simulink model "AOCS_FDIR"  (R2020b)
settings: Solver=ode45  StartTime=0.0  StopTime=200  FixedStep=1e-4  MaxStep=0.25  RelTol=1e-8  AbsTol=1e-8
values from neighbouring files (symbols this model uses):
  Gyros = zeros(3,6)    [Generate_Data.m]
  ReWhe = zeros(3,4)    [Generate_Data.m]
  Thrus = ones(1,8)    [Generate_Data.m]
undefined symbols (not defined in the file or in its folder): A, A_FEEP, A_FEEP_real, A_mag, CG_real, d_face, Dipole_SC, e0_0, e1_0, e2_0, e3_0, e_max_att, e_max_orb, Env_Drag, Env_J2, Env_Moon, Env_Sun, Env_TGG, Env_TMag, FEEP, g, GNSS, gyr, h_ref, h_RW, h_rw_0, I, I_real, IAU, initial_date_JD, J2, K_det, k_quat, km, m, mag, mu, mu_Moon, mu_Sun, n, n_orbits, q_0, Re, RW1, RW2, RW3, RW4, rx0, ry0, rz0, s, sigma1, sigma2, star, T_friction, th_2_gyr, th_FR_gyr, th_RW, th_SD_gyr_null, th_thruster ... (+10)
libraries: dspstat3 x16, aerolibutil x8, sharedutil x6, sharedtransform x5, vrlib x3, aerolibtransform2 x3, aerolibcelestial x2, aerolibobsolete x1, dspinverses x1
(part 1 of 4)
settings Model: PacingRate=1000  Creator=JavierSanzLobo  LastModifiedBy=Pepe
settings SolverCC: AutoScaleAbsTol=off  ShapePreserveControl=EnableAll  ZeroCrossControl=DisableAll  ZeroCrossAlgorithm=Adaptive  AutoInsertRateTranBlk=on  DecoupledContinuousIntegration=on  MinimalZcImpactIntegration=on
settings DataIOCC: ReturnWorkspaceOutputs=off
settings DebuggingCC: ArithmeticOperatorsInVariantConditions=warning
settings SFSimCC: SimUseLocalCustomCode=off  CustomCodeUndefinedFunction=UseInterfaceOnly
settings RTWCC: RTWUseLocalCustomCode=off

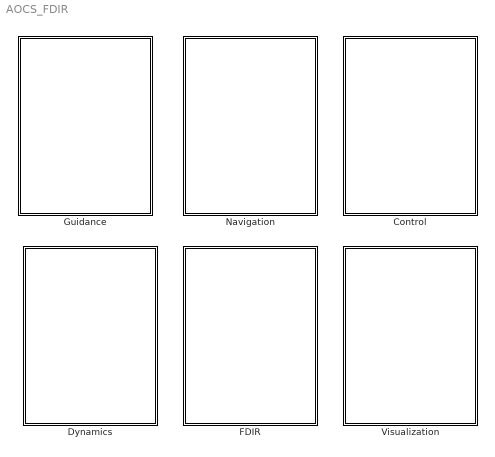
== system AOCS_FDIR ==
  Control : Subsystem
  Dynamics : Subsystem
  FDIR : Subsystem
  Guidance : Subsystem
  Navigation : Subsystem
  Visualization : Subsystem

== system AOCS_FDIR/Control ==
  Attitude Control : Subsystem
  Orbit Control : Subsystem

== system AOCS_FDIR/Dynamics ==
  6DOF Model : Subsystem
  Add : Sum  Inputs=+++
  Add1 : Sum
  Add2 : Sum  Inputs=+++
  Demux : Demux  Outputs=3
  Environmet : Subsystem
  Gain : Gain  Gain=180/pi
  "Keplerian Orbit " : Subsystem
  Scope1 : Scope  NumInputPorts=3
  tag scope: q_b_ECI=global, r=global, v=global, wb=global
  wires:
  Environmet/1(a_Env) -> Add/2
  "Keplerian Orbit "/1(a_kep) -> Add/1
  Add/1 -> 6DOF Model/1(a_ECI)  "Acceleration"
  6DOF Model/1("r_ECI ") -> [r], "Keplerian Orbit "/1(r), Environmet/1(r)  "Position"
  6DOF Model/2(v_ECI) -> [v], Environmet/2(v)  "Velocity"
  6DOF Model/4(q_b/ECI) -> Environmet/3(q_b/ECI), [q_b_ECI]
  6DOF Model/5(Euler_b/LVLH) -> Gain/1
  Demux/2 -> Scope1/2  "Pitch"
  Gain/1 -> Demux/1
  Demux/1 -> Scope1/1  "Roll"
  Demux/3 -> Scope1/3  "Yaw"
  [a_F] -> Add/3  "Orbit Control"
  6DOF Model/3(p q r) -> [wb]  "Angular Speed"
  Environmet/2(T_Env) -> Add1/1
  Add1/1 -> 6DOF Model/2(M_body)  "Moments"
  Add2/1 -> Add1/2  "Attitude Control"
  [T_rw] -> Add2/1
  [T_F] -> Add2/3
  [T_mt] -> Add2/2

== system AOCS_FDIR/FDIR ==
  Gyroscopes FDIR : Subsystem
  Reaction Wheels FDIR : Subsystem
  Thrusters FDIR : Subsystem

== system AOCS_FDIR/Guidance ==
  note: Earth Pointing
  note: Nominal Orbit
  Constant : Constant  Value=mu
  Constant1 : Constant  Value=[0; 0; -2*pi/(24*3600/n_orbits)]
  Direction Cosine Matrix to Quaternions : sharedtransform/Direction Cosine Matrix  to Quaternions  aMode=0  action=None  tolerance=eps(2)
      settings: SourceProductBaseCode=AE,PW,MT,UV,VE,VP
  Divide : Product  Inputs=*/
  Dot Product : DotProduct  InputSameDT=on  OutDataTypeStr=Inherit: Inherit via internal rule
  Gain : Gain  Gain=-1
  Integrator : Integrator  InitialCondition=[vx0, vy0, vz0]
  Integrator1 : Integrator  InitialCondition=[rx0, ry0, rz0]
  MATLAB Function1 : MATLAB Function  TreatAsAtomicUnit=on
  Normalize Vector : vrlib/Utilities/Normalize Vector  maxzero=0
  Product : Product
  To File1 : ToFile  Commented=on  Filename=r_des.mat  MatrixName=r_des
  To File2 : ToFile  Commented=on  Filename=v_des.mat  MatrixName=v_des
  To File3 : ToFile  Commented=on  Filename=q_des.mat  MatrixName=q_des
  tag scope: q_des=global, r_des=global, v_des=global, wb_des=global
  wires:
  Constant/1 -> Gain/1
  Gain/1 -> Divide/1
  Dot Product/1 -> Divide/2
  Divide/1 -> Product/1
  Product/1 -> Integrator/1  "Keplerian Acceleration"
  Integrator/1 -> Integrator1/1, [v_des], To File2/1  "Desired Speed"
  Integrator1/1 -> [r_des], To File1/1, Normalize Vector/1, Dot Product/2, Dot Product/1  "Desired Position"
  Normalize Vector/1 -> Product/2
  MATLAB Function1/1(DCM_Pointing_ECI) -> Direction Cosine Matrix to Quaternions/1
  [v_est] -> MATLAB Function1/2(v)
  [r_est] -> MATLAB Function1/1(r)
  Direction Cosine Matrix to Quaternions/1 -> To File3/1, [q_des]  "Attitude Desired (Earth pointing)"
  Constant1/1 -> [wb_des]  "Angular Speed Desired"

== system AOCS_FDIR/Navigation ==
  note: Attitude Estimation
  note: Orbit Estimation
  note: True states
  Add : Sum  Inputs=+-
  Attitude Filter : Subsystem
  GNSS : Subsystem
  Gyroscope : Subsystem
  Orbit Filter : Subsystem
  Scope : Scope  NumInputPorts=2
  Scope1 : Scope
  Star tracker : Subsystem
  To File2 : ToFile  Commented=on  Filename=Error_est.mat  MatrixName=Error_est
  tag scope: q_b_est=global, r_est=global, v_est=global, wb_est=global
  wires:
  [q_b_ECI] -> Star tracker/1(q_b_ECI)
  [r] -> GNSS/1(r)
  [v] -> GNSS/2(v)
  [wb] -> Gyroscope/1(wb), Scope/2, Add/1
  GNSS/1(r_GNSS) -> Orbit Filter/1(r_GNSS)
  GNSS/2(v_GNSS) -> Orbit Filter/2(v_GNSS)
  Orbit Filter/1(r_est) -> [r_est]
  Orbit Filter/2(v_est) -> [v_est]
  Add/1 -> Scope1/1, To File2/1
  Attitude Filter/1(wb_est) -> Add/2, [wb_est], Scope/1
  Attitude Filter/2(q_b_est) -> [q_b_est]
  Star tracker/1(q_b_star) -> Attitude Filter/2(q_b_star)
  Gyroscope/1(wb_gyr) -> Attitude Filter/1(wb_gyr)

== system AOCS_FDIR/Visualization ==
  3D Orbit : Subsystem  Commented=on
  COE : Subsystem
  Groundtrack : Subsystem  Commented=on

== system AOCS_FDIR/Control/Attitude Control ==
  Attitude Controller : Subsystem
  Magnetorquer : Subsystem
  Reaction Wheel Allocation : Subsystem
  Reaction Wheel Controller : Subsystem
  Reaction Wheel Model : Subsystem
  Scope : Scope
  Scope1 : Scope
  Scope3 : Scope
  To File1 : ToFile  Commented=on  Filename=T_rw.mat  MatrixName=T_rw
  To File2 : ToFile  Commented=on  Filename=h_rw_sum.mat  MatrixName=h_rw_sum
  To File3 : ToFile  Commented=on  Filename=T_mt.mat  MatrixName=T_mt
  tag scope: T_mt=global, T_rw=global, hrw=global
  wires:
  [q_b_est] -> Attitude Controller/3(q)  "Actual Attitude"
  [wb_est] -> Attitude Controller/4(wb)  "Actual angular speed"
  [q_des] -> Attitude Controller/1(q_des)  "Attitude Desired (Earth pointing)"
  [wb_des] -> Attitude Controller/2(wb_des)  "Angular Speed Desired"
  Attitude Controller/1(u_att) -> Reaction Wheel Controller/1(u_att)  "Torque Commanded"
  Reaction Wheel Model/1(T_rw) -> To File1/1, [T_rw], Scope/1
  Reaction Wheel Model/2(h_rw) -> To File2/1, [hrw], Scope1/1
  Reaction Wheel Controller/1(T_rw_c) -> Reaction Wheel Allocation/1(T_rw_c)
  Reaction Wheel Allocation/1(T_RW1_c) -> Reaction Wheel Model/1(T_RW1_c)
  Magnetorquer/1(T_mt) -> To File3/1, [T_mt], Scope3/1
  Reaction Wheel Allocation/2(T_RW2_c) -> Reaction Wheel Model/2(T_RW2_c)
  Reaction Wheel Allocation/3(T_RW3_c) -> Reaction Wheel Model/3(T_RW3_c)
  Reaction Wheel Allocation/4(T_RW4_c) -> Reaction Wheel Model/4(T_RW4_c)

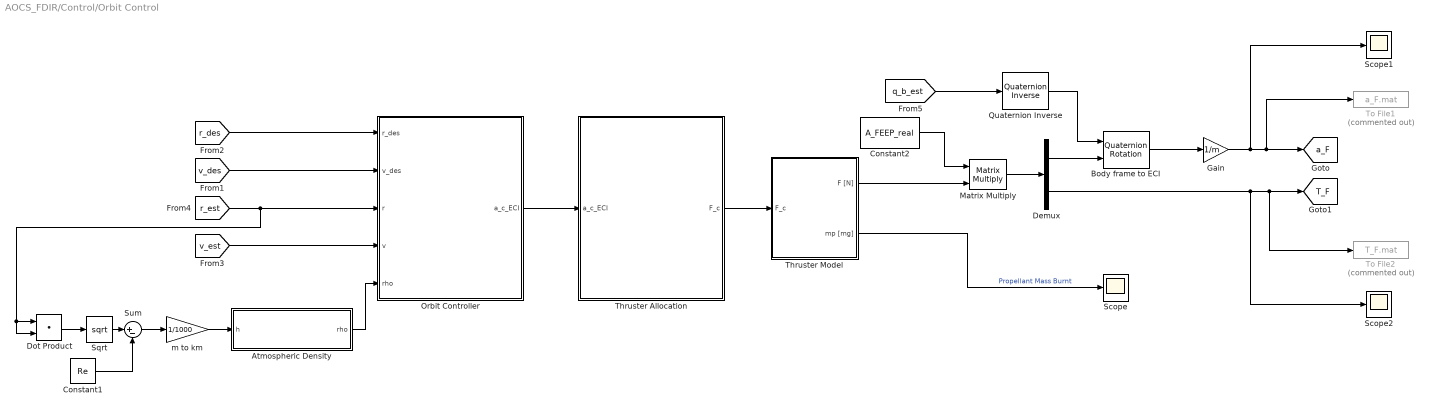
== system AOCS_FDIR/Control/Orbit Control ==
  Atmospheric Density : MATLAB Function  TreatAsAtomicUnit=on
  Body frame to ECI : aerolibutil/Quaternion Rotation
  Constant1 : Constant  Value=Re
  Constant2 : Constant  Value=A_FEEP_real
  Demux : Demux  Outputs=2
  Dot Product : DotProduct  InputSameDT=on  OutDataTypeStr=Inherit: Inherit via internal rule
  Gain : Gain  Gain=1/m
  Matrix Multiply : Product  Multiplication=Matrix(*)
  Orbit Controller : Subsystem
  Quaternion Inverse : aerolibutil/Quaternion Inverse
  Scope : Scope
  Scope1 : Scope
  Scope2 : Scope
  Sqrt : Sqrt  SaturateOnIntegerOverflow=on
  Sum : Sum  Inputs=|+-
  Thruster Allocation : Subsystem
  Thruster Model : Subsystem
  To File1 : ToFile  Commented=on  Filename=a_F.mat  MatrixName=a_F
  To File2 : ToFile  Commented=on  Filename=T_F.mat  MatrixName=T_F
  m to km : Gain  Gain=1/1000
  tag scope: T_F=global, a_F=global
  wires:
  [r_est] -> Dot Product/2, Dot Product/1, Orbit Controller/3(r)
  [v_est] -> Orbit Controller/4(v)
  Atmospheric Density/1(rho) -> Orbit Controller/5(rho)
  Dot Product/1 -> Sqrt/1
  Sqrt/1 -> Sum/1
  Sum/1 -> m to km/1
  Constant1/1 -> Sum/2
  m to km/1 -> Atmospheric Density/1(h)
  Orbit Controller/1(a_c_ECI) -> Thruster Allocation/1(a_c_ECI)
  Thruster Allocation/1(F_c) -> Thruster Model/1(F_c)
  Thruster Model/1(F [N]) -> Matrix Multiply/2
  Constant2/1 -> Matrix Multiply/1
  Matrix Multiply/1 -> Demux/1
  Gain/1 -> To File1/1, [a_F], Scope1/1
  Demux/2 -> To File2/1, [T_F], Scope2/1
  Thruster Model/2(mp [mg]) -> Scope/1  "Propellant Mass Burnt"
  Quaternion Inverse/1 -> Body frame to ECI/1
  [q_b_est] -> Quaternion Inverse/1
  Demux/1 -> Body frame to ECI/2
  Body frame to ECI/1 -> Gain/1
  [r_des] -> Orbit Controller/1(r_des)
  [v_des] -> Orbit Controller/2(v_des)

== system AOCS_FDIR/Dynamics/6DOF Model ==
  a_ECI : Inport
  M_body : Inport  Port=2
  Attitude Dynamics : Subsystem
  Attitude Kinematics : Subsystem
  ECI to body frame : aerolibutil/Quaternion Rotation
  Integrator : Integrator  InitialCondition=[vx0, vy0, vz0]
  Integrator1 : Integrator  InitialCondition=[rx0, ry0, rz0]
  Terminator : Terminator
  Terminator2 : Terminator
  Terminator3 : Terminator
  To File1 : ToFile  Commented=on  Filename=r.mat  MatrixName=r
  To File2 : ToFile  Commented=on  Filename=v.mat  MatrixName=v
  To File3 : ToFile  Commented=on  Filename=q_b.mat  MatrixName=q_b
  To File4 : ToFile  Commented=on  Filename=Euler.mat  MatrixName=Euler
  To File5 : ToFile  Commented=on  Filename=wb.mat  MatrixName=wb
  "r_ECI " : Outport  VectorParamsAs1DForOutWhenUnconnected=off
  v_ECI : Outport  Port=2  VectorParamsAs1DForOutWhenUnconnected=off
  p q r : Outport  Port=3  VectorParamsAs1DForOutWhenUnconnected=off
  q_b/ECI : Outport  Port=4  VectorParamsAs1DForOutWhenUnconnected=off
  Euler_b/LVLH : Outport  Port=5  VectorParamsAs1DForOutWhenUnconnected=off
  tag scope: DCM_ECI=global
  wires:
  Integrator1/1 -> To File1/1, "r_ECI "/1
  Integrator/1 -> To File2/1, v_ECI/1, Integrator1/1
  M_body/1 -> Attitude Dynamics/1(M_body)
  Attitude Dynamics/1("p q r ") -> To File5/1, p q r/1, Attitude Kinematics/1(p q r)
  Attitude Kinematics/1(Euler_b/ECI) -> Terminator/1
  Attitude Kinematics/2(DCM_b/ECI) -> [DCM_ECI]
  Attitude Kinematics/3(q_b/ECI) -> ECI to body frame/1, To File3/1, q_b/ECI/1
  Attitude Kinematics/4(Euler_b/LVLH) -> To File4/1, Euler_b/LVLH/1
  a_ECI/1 -> ECI to body frame/2, Integrator/1
  Attitude Dynamics/2("pdot qdot rdot ") -> Terminator3/1
  ECI to body frame/1 -> Terminator2/1  "Body Acceleration"

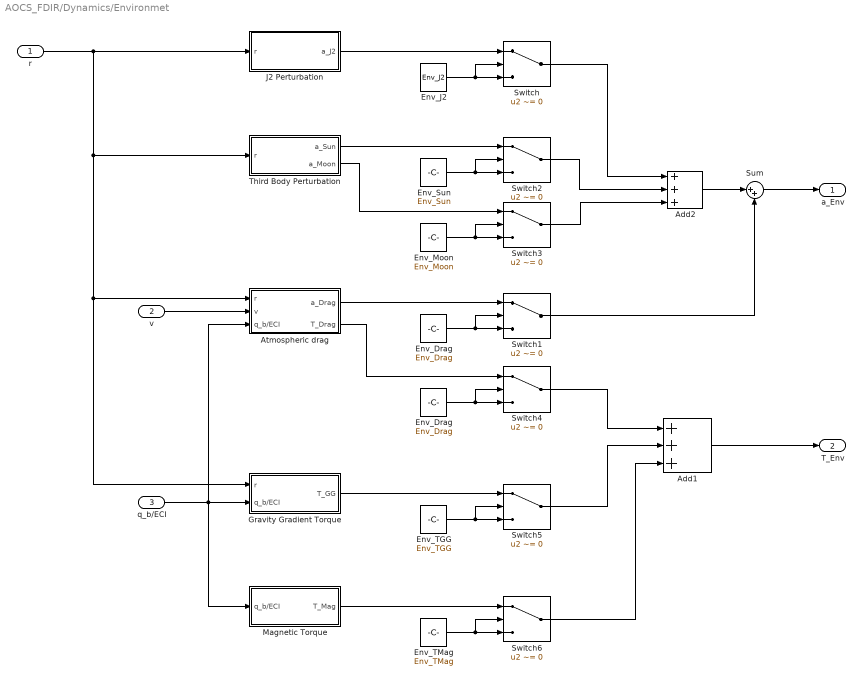
== system AOCS_FDIR/Dynamics/Environmet ==
  r : Inport
  v : Inport  Port=2
  q_b/ECI : Inport  Port=3
  Add1 : Sum  Inputs=+++
  Add2 : Sum  Inputs=+++
  Atmospheric drag : Subsystem
  "Env_Drag " : Constant  Value=Env_Drag
  "Env_Drag " : Constant  Value=Env_Drag
  "Env_J2 " : Constant  Value=Env_J2
  "Env_Moon " : Constant  Value=Env_Moon
  "Env_Sun " : Constant  Value=Env_Sun
  Env_TGG : Constant  Value=Env_TGG
  Env_TMag : Constant  Value=Env_TMag
  Gravity Gradient Torque : Subsystem
  "J2 Perturbation " : Subsystem
  Magnetic Torque : Subsystem
  Sum : Sum  Inputs=|++
  Switch{,1..6} (7 alike) : Switch  Criteria=u2 ~= 0
  Third Body Perturbation : Subsystem
  a_Env : Outport  VectorParamsAs1DForOutWhenUnconnected=off
  T_Env : Outport  Port=2  VectorParamsAs1DForOutWhenUnconnected=off
  wires:
  v/1 -> Atmospheric drag/2(v)
  r/1 -> "J2 Perturbation "/1(r), Third Body Perturbation/1(r), Atmospheric drag/1(r), Gravity Gradient Torque/1("r ")
  "J2 Perturbation "/1(a_J2) -> Switch/1
  "Env_J2 "/1 -> Switch/3, Switch/2
  Atmospheric drag/1(a_Drag) -> Switch1/1
  "Env_Drag "/1 -> Switch1/3, Switch1/2
  Third Body Perturbation/1(a_Sun) -> Switch2/1
  "Env_Sun "/1 -> Switch2/3, Switch2/2
  "Env_Moon "/1 -> Switch3/3, Switch3/2
  Third Body Perturbation/2(a_Moon) -> Switch3/1
  Switch1/1 -> Sum/2
  Switch/1 -> Add2/1
  Switch2/1 -> Add2/2
  Switch3/1 -> Add2/3
  q_b/ECI/1 -> Magnetic Torque/1(q_b/ECI), Atmospheric drag/3("q_b/ECI "), Gravity Gradient Torque/2("q_b/ECI ")
  Atmospheric drag/2(T_Drag) -> Switch4/1
  "Env_Drag "/1 -> Switch4/3, Switch4/2
  Env_TGG/1 -> Switch5/3, Switch5/2
  Gravity Gradient Torque/1(T_GG) -> Switch5/1
  Switch5/1 -> Add1/2
  Switch4/1 -> Add1/1
  Add1/1 -> T_Env/1
  Env_TMag/1 -> Switch6/3, Switch6/2
  Magnetic Torque/1(T_Mag) -> Switch6/1
  Switch6/1 -> Add1/3
  Add2/1 -> Sum/1
  Sum/1 -> a_Env/1

== system AOCS_FDIR/Dynamics/Keplerian Orbit  ==
  r : Inport
  Constant : Constant  Value=mu
  Divide : Product  Inputs=*/
  Dot Product : DotProduct  InputSameDT=on  OutDataTypeStr=Inherit: Inherit via internal rule
  Gain : Gain  Gain=-1
  Normalize Vector : vrlib/Utilities/Normalize Vector  maxzero=0
  Product : Product
  a_kep : Outport  VectorParamsAs1DForOutWhenUnconnected=off
  wires:
  Normalize Vector/1 -> Product/2
  r/1 -> Normalize Vector/1, Dot Product/2, Dot Product/1
  Constant/1 -> Gain/1
  Product/1 -> a_kep/1
  Divide/1 -> Product/1
  Gain/1 -> Divide/1
  Dot Product/1 -> Divide/2

== system AOCS_FDIR/FDIR/Gyroscopes FDIR ==
  Failure Control Panel : Subsystem
  Level 1 : Subsystem
  Level 2 : Subsystem

== system AOCS_FDIR/FDIR/Reaction Wheels FDIR ==
  Failure Control Panel : Subsystem
  RW Diagnosis : Subsystem

== system AOCS_FDIR/FDIR/Thrusters FDIR ==
  Failure Control Panel : Subsystem
  Thruster Diagnosis : Subsystem

== system AOCS_FDIR/Navigation/Attitude Filter ==
  wb_gyr : Inport
  q_b_star : Inport  Port=2
  Constant : Constant  Value=gyr.rate
  Constant1 : Constant  Value=gyr.ARW
  Constant2 : Constant  Value=gyr.RRW
  Constant3 : Constant  Value=star.accu
  Constant4 : Constant  Value=q_0
  Constant5 : Constant  Value=gyr.bias
  Constant6 : Constant  Value=gyr.H
  MATLAB Function : MATLAB Function  TreatAsAtomicUnit=on  SystemSampleTime=gyr.rate
  Pulse Generator : DiscretePulseGenerator  PulseType=Time based  Period=star.rate  PulseWidth=0.01
  To File1 : ToFile  Commented=on  Filename=q_b_est.mat  MatrixName=q_b_est
  To File2 : ToFile  Commented=on  Filename=wb_est.mat  MatrixName=wb_est
  wb_est : Outport  VectorParamsAs1DForOutWhenUnconnected=off
  q_b_est : Outport  Port=2  VectorParamsAs1DForOutWhenUnconnected=off
  tag scope: Pk1=global
  wires:
  Constant/1 -> MATLAB Function/5(dt)
  Constant1/1 -> MATLAB Function/6(ARW)
  Constant2/1 -> MATLAB Function/7(RRW)
  Constant3/1 -> MATLAB Function/8(sig_st)
  Pulse Generator/1 -> MATLAB Function/9(mflag)
  Constant4/1 -> MATLAB Function/3(q_0)
  Constant5/1 -> MATLAB Function/4(bias_0)
  MATLAB Function/3(Pk1) -> [Pk1]
  wb_gyr/1 -> MATLAB Function/1(wk1t)
  q_b_star/1 -> MATLAB Function/2(yk1)
  MATLAB Function/1(wk1) -> wb_est/1, To File2/1
  MATLAB Function/2(qk1) -> q_b_est/1, To File1/1
  Constant6/1 -> MATLAB Function/10(gyr_H)

== system AOCS_FDIR/Navigation/GNSS ==
  r : Inport
  v : Inport  Port=2
  Add : Sum
  Add1 : Sum
  Random Number : RandomNumber  Variance=GNSS.pos.^2  Seed=[23341 23342 23343]
  Random Number1 : RandomNumber  Variance=GNSS.vel.^2  Seed=[24341 24342 24343]
  Rate Transition1 : RateTransition  InitialCondition=[rx0;ry0;rz0]  OutPortSampleTime=GNSS.rate
  Rate Transition2 : RateTransition  InitialCondition=[vx0;vy0;vz0]  OutPortSampleTime=GNSS.rate
  To File1 : ToFile  Commented=on  Filename=v_GNSS.mat  MatrixName=v_GNSS
  To File2 : ToFile  Commented=on  Filename=r_GNSS.mat  MatrixName=r_GNSS
  r_GNSS : Outport  VectorParamsAs1DForOutWhenUnconnected=off
  v_GNSS : Outport  Port=2  VectorParamsAs1DForOutWhenUnconnected=off
  wires:
  Random Number/1 -> Add/1
  Add/1 -> Rate Transition1/1
  Add1/1 -> Rate Transition2/1
  Random Number1/1 -> Add1/2
  r/1 -> Add/2
  v/1 -> Add1/1
  Rate Transition1/1 -> To File2/1, r_GNSS/1
  Rate Transition2/1 -> To File1/1, v_GNSS/1

== system AOCS_FDIR/Navigation/Gyroscope ==
  wb : Inport
  Gyroscope Model : Subsystem
  wb_gyr : Outport  VectorParamsAs1DForOutWhenUnconnected=off
  tag scope: wb_gyr=global
  wires:
  wb/1 -> Gyroscope Model/1(wb)
  Gyroscope Model/1(wb_gyr) -> [wb_gyr], wb_gyr/1

== system AOCS_FDIR/Navigation/Orbit Filter ==
  r_GNSS : Inport
  v_GNSS : Inport  Port=2
  Constant : Constant  Value=GNSS.rate
  Constant1 : Constant  Value=GNSS.pos
  Constant2 : Constant  Value=GNSS.vel
  MATLAB Function : MATLAB Function  TreatAsAtomicUnit=on
  Mux : Mux  Inputs=2
  To File1 : ToFile  Commented=on  Filename=v_est.mat  MatrixName=v_est
  To File2 : ToFile  Commented=on  Filename=r_est.mat  MatrixName=r_est
  r_est : Outport  VectorParamsAs1DForOutWhenUnconnected=off
  v_est : Outport  Port=2  VectorParamsAs1DForOutWhenUnconnected=off
  wires:
  r_GNSS/1 -> Mux/1
  MATLAB Function/2(vk1) -> v_est/1, To File1/1
  Constant/1 -> MATLAB Function/2(dt)
  Constant1/1 -> MATLAB Function/3(sig_r)
  v_GNSS/1 -> Mux/2
  Constant2/1 -> MATLAB Function/4(sig_v)
  Mux/1 -> MATLAB Function/1(z)
  MATLAB Function/1(rk1) -> To File2/1, r_est/1

== system AOCS_FDIR/Navigation/Star tracker ==
  q_b_ECI : Inport
  Quaternion Multiplication : aerolibutil/Quaternion Multiplication
  Random Number : RandomNumber  Variance=star.accu.^2  Seed=[20341 20342 20343]
  Rate Transition : RateTransition  InitialCondition=q_0  OutPortSampleTime=star.rate
  Rotation Angles to Quaternions : sharedtransform/Rotation Angles to Quaternions  rotationOrder=ZYX  aMode=aMode
      settings: SourceProductBaseCode=AE,PW,MT,UV,VE,VP
  Scope : Scope
  Selector : Selector  InputPortWidth=3  IndexOptions=Index vector (dialog)  Indices=[3 2 1]  OutputSizes=1
  To File2 : ToFile  Commented=on  Filename=q_b_star.mat  MatrixName=q_b_star
  q_b_star : Outport  VectorParamsAs1DForOutWhenUnconnected=off
  wires:
  q_b_ECI/1 -> Scope/1, Quaternion Multiplication/1
  Random Number/1 -> Selector/1  "Angle Noise"
  Selector/1 -> Rotation Angles to Quaternions/1
  Rotation Angles to Quaternions/1 -> Quaternion Multiplication/2  "Quaternion Noise"
  Quaternion Multiplication/1 -> Rate Transition/1
  Rate Transition/1 -> To File2/1, q_b_star/1

== system AOCS_FDIR/Visualization/3D Orbit ==
  3D Orbit Plot : MATLAB Function  TreatAsAtomicUnit=on  SystemSampleTime=100
  Clock : Clock
  wires:
  Clock/1 -> 3D Orbit Plot/4(time)
  [DCM_ECI] -> 3D Orbit Plot/3(DCM)
  [v] -> 3D Orbit Plot/2(v)
  [r] -> 3D Orbit Plot/1(x)

== system AOCS_FDIR/Visualization/COE ==
  From1 : From  Commented=on  GotoTag=v_des  TagVisibility=global
  From2 : From  Commented=on  GotoTag=r_des  TagVisibility=global
  MATLAB Function : MATLAB Function  Commented=on  TreatAsAtomicUnit=on
  MATLAB Function1 : MATLAB Function  TreatAsAtomicUnit=on
  "Orbit " : Scope  NumInputPorts=6
  "Orbit Desired " : Scope  Commented=on  NumInputPorts=6
  wires:
  From2/1 -> MATLAB Function/1(R)
  MATLAB Function/6(TA) -> "Orbit Desired "/6
  MATLAB Function/4(RA) -> "Orbit Desired "/4
  MATLAB Function/3(i) -> "Orbit Desired "/3
  From1/1 -> MATLAB Function/2(V)
  MATLAB Function/5(w) -> "Orbit Desired "/5
  MATLAB Function/2(e) -> "Orbit Desired "/2
  MATLAB Function/1(a) -> "Orbit Desired "/1
  MATLAB Function1/4(RA) -> "Orbit "/4
  MATLAB Function1/6(TA) -> "Orbit "/6
  MATLAB Function1/5(w) -> "Orbit "/5
  MATLAB Function1/1(a) -> "Orbit "/1
  [r] -> MATLAB Function1/1(R)
  MATLAB Function1/2(e) -> "Orbit "/2
  [v] -> MATLAB Function1/2(V)
  MATLAB Function1/3(i) -> "Orbit "/3

== system AOCS_FDIR/Visualization/Groundtrack ==
  Groundtrack : MATLAB Function  TreatAsAtomicUnit=on  SystemSampleTime=100
  wires:
  [lat] -> Groundtrack/1(lat)
  [lon] -> Groundtrack/2(lon)

== system AOCS_FDIR/Control/Attitude Control/Attitude Controller ==
  q_des : Inport
  wb_des : Inport  Port=2
  q : Inport  Port=3
  wb : Inport  Port=4
  Demux : Demux  Outputs=3
  Inertia Matrix : Constant  Value=I
  MATLAB Function1 : MATLAB Function  TreatAsAtomicUnit=on  SystemSampleTime=gyr.rate
  Max. Control Input : Constant  Value=u_max_att
  Max. Error Allowed : Constant  Value=e_max_att
  Scope : Scope  NumInputPorts=3
  To File1 : ToFile  Commented=on  Filename=u_att.mat  MatrixName=u_att
  u_att : Outport  VectorParamsAs1DForOutWhenUnconnected=off
  tag scope: u_att=global
  wires:
  q_des/1 -> MATLAB Function1/1(q_des)
  wb_des/1 -> MATLAB Function1/2(wb_des)
  q/1 -> MATLAB Function1/3(q)
  wb/1 -> MATLAB Function1/4(wb)
  Inertia Matrix/1 -> MATLAB Function1/5(I)
  MATLAB Function1/1(u_att) -> Demux/1, [u_att], u_att/1, To File1/1
  Max. Error Allowed/1 -> MATLAB Function1/6(e_max_att)
  Max. Control Input/1 -> MATLAB Function1/7(u_max_att)
  Demux/1 -> Scope/1
  Demux/2 -> Scope/2
  Demux/3 -> Scope/3

== system AOCS_FDIR/Control/Attitude Control/Magnetorquer ==
  note: Magnetorquer Modelling
  3x3 Cross Product : sharedutil/3x3 Cross Product  aMode=aMode
      settings: SourceProductBaseCode=AE,PW,MT,UV,VE,VP
  Add : Sum
  Add1 : Sum
  Add2 : Sum
  Constant : Constant  Value=A_mag
  Demux : Demux  Outputs=6
  Matrix Divide : Product  Inputs=*/  Multiplication=Matrix(*)
  Matrix Multiply : Product  Multiplication=Matrix(*)
  Mux : Mux  Inputs=3
  Product : Product  Multiplication=Matrix(*)
  Product1 : Product
  Quantizer : Quantizer  QuantizationInterval=2*mag.sat/(2^mag.bits-1)
  Saturation : Saturate  UpperLimit=ones(6,1)*mag.sat  LowerLimit=-ones(6,1)*mag.sat
  Scope : Scope
  To File3 : ToFile  Commented=on  Filename=m_mt.mat  MatrixName=m_mt
  Transpose : Math  Operator=transpose  SignedPower=on  SaturateOnIntegerOverflow=on
  Uniform Random Number2 : UniformRandomNumber  Minimum=(100-mag.error/3)/100  Maximum=(100+mag.error/3)/100  Seed=[30 31 32 33 34 35]
  Update Rate : RateTransition  InitialCondition=zeros(6,1)  OutPortSampleTime=mag.rate
  T_mt : Outport  VectorParamsAs1DForOutWhenUnconnected=off
  wires:
  [m_mt_c] -> Product/2
  Matrix Divide/1 -> Product/1  "Pseudo-Inverse"
  Transpose/1 -> Matrix Multiply/2, Matrix Divide/1
  Matrix Multiply/1 -> Matrix Divide/2
  Constant/1 -> Transpose/1, Matrix Multiply/1  "Configuration Matrix"
  Product/1 -> Product1/1
  Uniform Random Number2/1 -> Product1/2
  Product1/1 -> Update Rate/1
  Demux/1 -> Add/1
  Demux/2 -> Add/2
  Demux/3 -> Add1/1
  Demux/4 -> Add1/2
  Demux/5 -> Add2/1
  Demux/6 -> Add2/2
  Add/1 -> Mux/1
  Add1/1 -> Mux/2
  Add2/1 -> Mux/3
  Mux/1 -> Scope/1, 3x3 Cross Product/1
  3x3 Cross Product/1 -> T_mt/1
  [B_b] -> 3x3 Cross Product/2
  Saturation/1 -> To File3/1, Demux/1
  Quantizer/1 -> Saturation/1
  Update Rate/1 -> Quantizer/1

== system AOCS_FDIR/Control/Attitude Control/Reaction Wheel Allocation ==
  T_rw_c : Inport
  Constant : Constant  Value=RW1.pos
  Constant1 : Constant  Value=RW2.pos
  Constant2 : Constant  Value=RW3.pos
  Constant3 : Constant  Value=RW4.pos
  Demux : Demux
  Matrix Divide : Product  Inputs=*/  Multiplication=Matrix(*)
  Matrix Multiply : Product  Multiplication=Matrix(*)
  Product : Product  Multiplication=Matrix(*)
  Recovery : MATLAB Function  TreatAsAtomicUnit=on
  Transpose : Math  Operator=transpose  SignedPower=on  SaturateOnIntegerOverflow=on
  T_RW1_c : Outport  VectorParamsAs1DForOutWhenUnconnected=off
  T_RW2_c : Outport  Port=2  VectorParamsAs1DForOutWhenUnconnected=off
  T_RW3_c : Outport  Port=3  VectorParamsAs1DForOutWhenUnconnected=off
  T_RW4_c : Outport  Port=4  VectorParamsAs1DForOutWhenUnconnected=off
  wires:
  T_rw_c/1 -> Product/2
  Product/1 -> Demux/1
  Matrix Divide/1 -> Product/1  "Pseudo-Inverse"
  Recovery/1(A_rw) -> Transpose/1, Matrix Multiply/1  "Configuration Matrix"
  Transpose/1 -> Matrix Multiply/2, Matrix Divide/1
  Matrix Multiply/1 -> Matrix Divide/2
  Demux/1 -> T_RW1_c/1
  Demux/2 -> T_RW2_c/1
  Demux/3 -> T_RW3_c/1
  Demux/4 -> T_RW4_c/1
  Constant/1 -> Recovery/1(RW1)
  Constant1/1 -> Recovery/2(RW2)
  Constant2/1 -> Recovery/3(RW3)
  Constant3/1 -> Recovery/4(RW4)
  [flagRW1] -> Recovery/5(flagRW1)
  [flagRW2] -> Recovery/6(flagRW2)
  [flagRW3] -> Recovery/7(flagRW3)
  [flagRW4] -> Recovery/8(flagRW4)

== system AOCS_FDIR/Control/Attitude Control/Reaction Wheel Controller ==
  u_att : Inport
  3x3 Cross Product : sharedutil/3x3 Cross Product  aMode=aMode
      settings: SourceProductBaseCode=AE,PW,MT,UV,VE,VP
  Add1 : Sum
  Gain : Gain  Gain=-1
  Gain1 : Gain  Gain=-1
  Gain3 : Gain  Gain=-1
  Integrator : Integrator  InitialCondition=h_rw_0
  Scope : Scope
  T_rw_c : Outport  VectorParamsAs1DForOutWhenUnconnected=off
  wires:
  u_att/1 -> Gain/1
  Gain/1 -> Add1/1
  [wb_est] -> 3x3 Cross Product/1
  3x3 Cross Product/1 -> Gain1/1
  Gain1/1 -> Add1/2
  Add1/1 -> Gain3/1, Integrator/1  "hrw_dot"
  Integrator/1 -> Scope/1, 3x3 Cross Product/2  "hrw_c"
  Gain3/1 -> T_rw_c/1

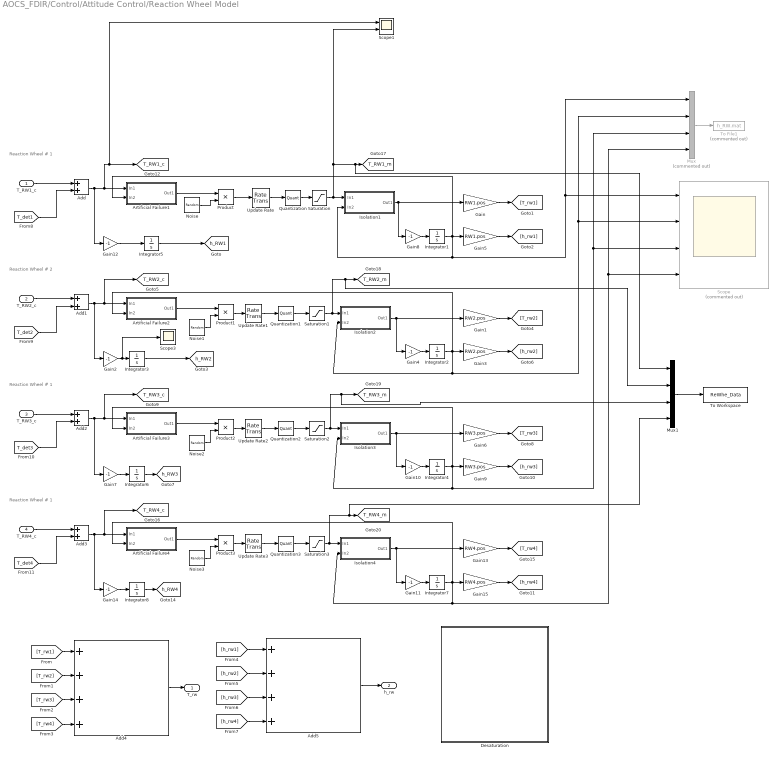
== system AOCS_FDIR/Control/Attitude Control/Reaction Wheel Model ==
  note: Reaction Wheel # 1
  note: Reaction Wheel # 2
  note: Reaction Wheel # 1
  note: Reaction Wheel # 1
  T_RW1_c : Inport
  T_RW2_c : Inport  Port=2
  T_RW3_c : Inport  Port=3
  T_RW4_c : Inport  Port=4
  Add{,1..3} (4 alike) : Sum
  Add4 : Sum  Inputs=++++
  Add5 : Sum  Inputs=++++
  Artificial Failure1 : Subsystem
  Artificial Failure2 : Subsystem
  Artificial Failure3 : Subsystem
  Artificial Failure4 : Subsystem
  Desaturation : Subsystem
  Gain : Gain  Gain=RW1.pos
  Gain1 : Gain  Gain=RW2.pos
  Gain{2,4,7..8,10..12,14} (8 alike) : Gain  Gain=-1
  Gain13 : Gain  Gain=RW4.pos
  Gain15 : Gain  Gain=RW4.pos
  Gain3 : Gain  Gain=RW2.pos
  Gain5 : Gain  Gain=RW1.pos
  Gain6 : Gain  Gain=RW3.pos
  Gain9 : Gain  Gain=RW3.pos
  Integrator1 : Integrator  InitialCondition=h_RW(1)
  Integrator2 : Integrator  InitialCondition=h_RW(2)
  Integrator3 : Integrator  InitialCondition=h_RW(2)
  Integrator4 : Integrator  InitialCondition=h_RW(3)
  Integrator5 : Integrator  InitialCondition=h_RW(2)
  Integrator6 : Integrator  InitialCondition=h_RW(3)
  Integrator7 : Integrator  InitialCondition=h_RW(4)
  Integrator8 : Integrator  InitialCondition=h_RW(4)
  Isolation1 : Subsystem
  Isolation2 : Subsystem
  Isolation3 : Subsystem
  Isolation4 : Subsystem
  Mux : Mux  Commented=on
  Mux1 : Mux
  Noise : UniformRandomNumber  Minimum=(100-RW1.error/3)/100  Maximum=(100+RW1.error/3)/100  Seed=451
  Noise1 : UniformRandomNumber  Minimum=(100-RW2.error/3)/100  Maximum=(100+RW2.error/3)/100  Seed=452
  Noise2 : UniformRandomNumber  Minimum=(100-RW3.error/3)/100  Maximum=(100+RW3.error/3)/100  Seed=453
  Noise3 : UniformRandomNumber  Minimum=(100-RW4.error/3)/100  Maximum=(100+RW4.error/3)/100  Seed=454
  Product{,1..3} (4 alike) : Product
  Quantization : Quantizer  QuantizationInterval=2*RW1.torque/(2^RW1.bits-1)
  Quantization1 : Quantizer  QuantizationInterval=2*RW2.torque/(2^RW2.bits-1)
  Quantization2 : Quantizer  QuantizationInterval=2*RW3.torque/(2^RW3.bits-1)
  Quantization3 : Quantizer  QuantizationInterval=2*RW4.torque/(2^RW4.bits-1)
  Saturation : Saturate  UpperLimit=RW1.torque  LowerLimit=-RW1.torque
  Saturation1 : Saturate  UpperLimit=RW2.torque  LowerLimit=-RW2.torque
  Saturation2 : Saturate  UpperLimit=RW3.torque  LowerLimit=-RW3.torque
  Saturation3 : Saturate  UpperLimit=RW4.torque  LowerLimit=-RW4.torque
  Scope : Scope  Commented=on  NumInputPorts=4
  Scope1 : Scope  NumInputPorts=2
  Scope3 : Scope
  To File1 : ToFile  Commented=on  Filename=h_RW.mat  MatrixName=h_RW
  To Workspace : ToWorkspace  VariableName=ReWhe_Data  SaveFormat=Timeseries  SampleTime=0.25
  Update Rate : RateTransition  OutPortSampleTime=RW1.rate
  Update Rate1 : RateTransition  OutPortSampleTime=RW2.rate
  Update Rate2 : RateTransition  OutPortSampleTime=RW3.rate
  Update Rate3 : RateTransition  OutPortSampleTime=RW4.rate
  T_rw : Outport  VectorParamsAs1DForOutWhenUnconnected=off
  h_rw : Outport  Port=2  VectorParamsAs1DForOutWhenUnconnected=off
  tag scope: T_RW1_c=global, T_RW1_m=global, T_RW2_c=global, T_RW2_m=global, T_RW3_c=global, T_RW3_m=global, T_RW4_c=global, T_RW4_m=global, h_RW1=global, h_RW2=global, h_RW3=global, h_RW4=global
  wires:
  Integrator1/1 -> Artificial Failure1/2(In2), Isolation1/2(In2), Mux/1, Scope/1, Gain5/1
  Gain8/1 -> Integrator1/1
  Gain/1 -> [T_rw1]
  Gain5/1 -> [h_rw1]
  [T_rw1] -> Add4/1
  [T_rw4] -> Add4/4
  [T_rw3] -> Add4/3
  [T_rw2] -> Add4/2
  Add4/1 -> T_rw/1
  Add5/1 -> h_rw/1
  [h_rw4] -> Add5/4
  [h_rw3] -> Add5/3
  [h_rw1] -> Add5/1
  [h_rw2] -> Add5/2
  Noise/1 -> Product/2
  Artificial Failure1/1(Out1) -> Product/1
  Add/1 -> Scope1/1, [T_RW1_c], Artificial Failure1/1(In1), Gain12/1
  T_RW1_c/1 -> Add/1
  [T_det1] -> Add/2
  Mux/1 -> To File1/1
  Update Rate/1 -> Quantization/1
  Product/1 -> Update Rate/1
  Quantization/1 -> Saturation/1
  Isolation1/1(Out1) -> Gain8/1, Gain/1
  Integrator3/1 -> [h_RW2]
  Product1/1 -> Update Rate1/1
  Quantization1/1 -> Saturation1/1
  Update Rate1/1 -> Quantization1/1
  Gain2/1 -> Scope3/1, Integrator3/1
  [T_det2] -> Add1/2
  Noise1/1 -> Product1/2
  Gain3/1 -> [h_rw2]
  Gain4/1 -> Integrator2/1
  Gain1/1 -> [T_rw2]
  Saturation1/1 -> Mux1/2, [T_RW2_m], Isolation2/1(In1)
  Integrator2/1 -> Artificial Failure2/2(In2), Isolation2/2(In2), Scope/2, Mux/2, Gain3/1
  Artificial Failure2/1(Out1) -> Product1/1
  T_RW2_c/1 -> Add1/1
  Isolation2/1(Out1) -> Gain4/1, Gain1/1
  Add1/1 -> [T_RW2_c], Artificial Failure2/1(In1), Gain2/1
  Integrator6/1 -> [h_RW3]
  Product2/1 -> Update Rate2/1
  Quantization2/1 -> Saturation2/1
  Update Rate2/1 -> Quantization2/1
  Gain7/1 -> Integrator6/1
  [T_det3] -> Add2/2
  Noise2/1 -> Product2/2
  Gain9/1 -> [h_rw3]
  Gain10/1 -> Integrator4/1
  Gain6/1 -> [T_rw3]
  Saturation2/1 -> Mux1/3, [T_RW3_m], Isolation3/1(In1)
  Integrator4/1 -> Artificial Failure3/2(In2), Isolation3/2(In2), Scope/3, Mux/3, Gain9/1
  Artificial Failure3/1(Out1) -> Product2/1
  T_RW3_c/1 -> Add2/1
  Isolation3/1(Out1) -> Gain10/1, Gain6/1
  Add2/1 -> [T_RW3_c], Artificial Failure3/1(In1), Gain7/1
  Add3/1 -> [T_RW4_c], Artificial Failure4/1(In1), Gain14/1
  Integrator7/1 -> Artificial Failure4/2(In2), Isolation4/2(In2), Scope/4, Mux/4, Gain15/1
  Isolation4/1(Out1) -> Gain11/1, Gain13/1
  T_RW4_c/1 -> Add3/1
  Artificial Failure4/1(Out1) -> Product3/1
  Saturation3/1 -> Mux1/4, [T_RW4_m], Isolation4/1(In1)
  Gain11/1 -> Integrator7/1
  Gain15/1 -> [h_rw4]
  Gain13/1 -> [T_rw4]
  [T_det4] -> Add3/2
  Noise3/1 -> Product3/2
  Gain14/1 -> Integrator8/1
  Quantization3/1 -> Saturation3/1
  Product3/1 -> Update Rate3/1
  Integrator8/1 -> [h_RW4]
  Update Rate3/1 -> Quantization3/1
  Saturation/1 -> Mux1/1, [T_RW1_m], Scope1/2, Isolation1/1(In1)
  Gain12/1 -> Integrator5/1
  Integrator5/1 -> [h_RW1]
  Mux1/1 -> To Workspace/1

== system AOCS_FDIR/Control/Orbit Control/Orbit Controller ==
  r_des : Inport
  v_des : Inport  Port=2
  r : Inport  Port=3
  v : Inport  Port=4
  rho : Inport  Port=5
  Constant : Constant  Value=mu
  Constant1 : Constant  Value=Re
  Constant2 : Constant  Value=J2
  Constant3 : Constant  Value=m
  MATLAB Function : MATLAB Function  TreatAsAtomicUnit=on  SystemSampleTime=GNSS.rate
  MATLAB Function1 : MATLAB Function  TreatAsAtomicUnit=on  SystemSampleTime=GNSS.rate
  MATLAB Function2 : MATLAB Function  TreatAsAtomicUnit=on  SystemSampleTime=1
  Max. Control Input : Constant  Value=u_max_orb
  Max. Error Allowed : Constant  Value=e_max_orb
  Scope : Scope
  Scope2 : Scope
  To File1 : ToFile  Commented=on  Filename=a_c_ECI.mat  MatrixName=a_c_ECI
  To File2 : ToFile  Commented=on  Filename=a_RSW.mat  MatrixName=a_RSW
  a_c_ECI : Outport  VectorParamsAs1DForOutWhenUnconnected=off
  wires:
  MATLAB Function1/4(RA) -> MATLAB Function2/10(RAAN)
  MATLAB Function/6(u) -> MATLAB Function2/6(u_N)
  Constant2/1 -> MATLAB Function2/15(J2)
  rho/1 -> MATLAB Function2/16(rho)
  MATLAB Function1/3(i) -> MATLAB Function2/9(i)
  MATLAB Function/5(w) -> MATLAB Function2/5(w_N)
  MATLAB Function1/2(e) -> MATLAB Function2/8(e)
  MATLAB Function/4(RA) -> MATLAB Function2/4(RAAN_N)
  MATLAB Function/2(e) -> MATLAB Function2/2(e_N)
  MATLAB Function1/1(a) -> MATLAB Function2/7(a)
  MATLAB Function1/5(w) -> MATLAB Function2/11(w)
  MATLAB Function/1(a) -> MATLAB Function2/1(a_N)
  Constant3/1 -> MATLAB Function2/17(m)
  Constant/1 -> MATLAB Function2/13(mu)
  Constant1/1 -> MATLAB Function2/14(Re)
  MATLAB Function/3(i) -> MATLAB Function2/3(i_N)
  MATLAB Function1/6(u) -> MATLAB Function2/12(u)
  v/1 -> MATLAB Function1/2(V)
  r/1 -> MATLAB Function1/1(R)
  Max. Error Allowed/1 -> MATLAB Function2/18(e_max_orb)
  Max. Control Input/1 -> MATLAB Function2/19(u_max_orb)
  v_des/1 -> MATLAB Function/2(V)
  r_des/1 -> MATLAB Function/1(R)
  MATLAB Function2/1(a_c) -> Scope2/1, To File1/1, a_c_ECI/1
  MATLAB Function2/2(a_RSW) -> To File2/1, Scope/1
  [n_thruster] -> MATLAB Function2/20(n_thruster)

== system AOCS_FDIR/Control/Orbit Control/Thruster Allocation ==
  a_c_ECI : Inport
  Constant : Constant  Value=m
  Constant1 : Constant  Value=[0;0;0]
  Constant2 : Constant  Value=A_FEEP
  ECI to body frame : aerolibutil/Quaternion Rotation
  Gain2 : Gain  Commented=on  Gain=1000000
  Isolation & Recovery : MATLAB Function  TreatAsAtomicUnit=on
  MATLAB Function : MATLAB Function  TreatAsAtomicUnit=on
  Max. Control Input : Constant  Commented=on  Value=FEEP.thrust
  Mux : Mux  Inputs=2
  N to microN : Gain  Gain=1000000
  Product : Product
  Scope : Scope
  Signal Specification : SignalSpecification  Dimensions=[6 8]
  Signal Specification1 : SignalSpecification  Dimensions=[8 1]
  To File1 : ToFile  Commented=on  Filename=F_T_b.mat  MatrixName=F_T_b
  F_c : Outport  VectorParamsAs1DForOutWhenUnconnected=off
  tag scope: firing=global
  wires:
  ECI to body frame/1 -> Product/1
  Constant/1 -> Product/2
  [q_b_est] -> ECI to body frame/1
  Max. Control Input/1 -> Gain2/1
  Product/1 -> Mux/1  "Thrust Desired"
  N to microN/1 -> To File1/1, MATLAB Function/1(F)
  Gain2/1 -> ?
  Mux/1 -> N to microN/1
  a_c_ECI/1 -> ECI to body frame/2
  MATLAB Function/1(F_thrusters) -> Signal Specification1/1
  Constant1/1 -> Mux/2
  MATLAB Function/2(firing) -> Scope/1, [firing]
  Constant2/1 -> Isolation & Recovery/1(A_FEEP)
  [flag_thruster] -> Isolation & Recovery/2(flag)
  Isolation & Recovery/1(y) -> Signal Specification/1
  Signal Specification/1 -> MATLAB Function/2(A_FEEP)
  Signal Specification1/1 -> F_c/1

== system AOCS_FDIR/Control/Orbit Control/Thruster Model ==
  note: Thruster Modelling
  F_c : Inport
  Add1 : Sum
  Artificial Failure : Subsystem
  Constant1 : Constant  Value=FEEP.quant*1000000
  Delay : UnitDelay  InitialCondition=zeros(8,1)  SampleTime=FEEP.rate  HasFrameUpgradeWarning=on
  Demux : Demux  Outputs=8
  Gain1 : Gain  Gain=1/sqrt(FEEP.rate)
  Gain2 : Gain  Gain=1/1000000
  Gravity Acceleration : Constant  Value=g
  Integrator : Integrator
  MATLAB Function : MATLAB Function  TreatAsAtomicUnit=on
  MATLAB Function1 : MATLAB Function  TreatAsAtomicUnit=on
  Noise : RandomNumber  Variance=(FEEP.noise*1000000).^2  Seed=[1;2;3;4;5;6;7;8]
  Product : Product
  Quantization : Quantizer  QuantizationInterval=FEEP.quant*1000000
  Response Limiter : RateLimiter  RisingSlewLimit=FEEP.response*1000000  FallingSlewLimit=-FEEP.response*1000000  SampleTimeMode=inherited  InitialCondition=zeros(8,1)
  Saturation : Saturate  UpperLimit=FEEP.thrust*ones(8,1)*1000000  LowerLimit=zeros(8,1)
  Scope : Scope  NumInputPorts=8
  Scope1 : Scope
  To File2 : ToFile  Commented=on  Filename=mp.mat  MatrixName=mp
  To Workspace : ToWorkspace  VariableName=Thrus_Data  SaveFormat=Timeseries  SampleTime=0.25
  Update Rate : RateTransition  InitialCondition=zeros(8,1)  OutPortSampleTime=FEEP.rate
  F [N] : Outport  VectorParamsAs1DForOutWhenUnconnected=off
  mp [mg] : Outport  Port=2  VectorParamsAs1DForOutWhenUnconnected=off
  wires:
  F_c/1 -> MATLAB Function1/1(F_des), Add1/1
  Demux/8 -> Scope/8  "# 8"
  Demux/7 -> Scope/7  "# 7"
  Demux/6 -> Scope/6  "# 6"
  Demux/5 -> Scope/5  "# 5"
  Demux/4 -> Scope/4  "# 4"
  Demux/3 -> Scope/3  "# 3"
  Demux/2 -> Scope/2  "# 2"
  Demux/1 -> Scope/1  "# 1"
  Gravity Acceleration/1 -> MATLAB Function/2(g)
  MATLAB Function/1(m_dot_p) -> Integrator/1
  Integrator/1 -> To File2/1, mp [mg]/1
  Gain2/1 -> F [N]/1
  Constant1/1 -> MATLAB Function1/2(quant)
  Product/1 -> Artificial Failure/1(In1)
  MATLAB Function1/1(y) -> Scope1/1, Product/2
  Saturation/1 -> Product/1
  Gain1/1 -> Add1/2
  Noise/1 -> Gain1/1
  Add1/1 -> Update Rate/1
  Update Rate/1 -> Quantization/1
  Quantization/1 -> Delay/1
  Delay/1 -> Response Limiter/1
  Response Limiter/1 -> Saturation/1
  Artificial Failure/1(Out1) -> To Workspace/1, Demux/1, MATLAB Function/1(F_c), Gain2/1

== system AOCS_FDIR/Dynamics/6DOF Model/Attitude Dynamics ==
  M_body : Inport
  " " : Integrator  InitialCondition=w_SC_0
  3x3 Cross Product : sharedutil/3x3 Cross Product  aMode=aMode
      settings: SourceProductBaseCode=AE,PW,MT,UV,VE,VP
  Add : Sum
  Inertia Matrix : Constant  Value=I_real
  Product : Product  Inputs=/  Multiplication=Matrix(*)
  Product1 : Product  Multiplication=Matrix(*)
  Product2 : Product  Multiplication=Matrix(*)
  Sum1 : Sum  Inputs=-+|
  "p q r " : Outport  VectorParamsAs1DForOutWhenUnconnected=off
  "pdot qdot rdot " : Outport  Port=2  VectorParamsAs1DForOutWhenUnconnected=off
  wires:
  Product/1 -> Product1/1
  Inertia Matrix/1 -> Product2/1, Product/1
  " "/1 -> "p q r "/1, 3x3 Cross Product/1, Product2/2
  M_body/1 -> Sum1/2
  3x3 Cross Product/1 -> Sum1/1
  Sum1/1 -> Product1/2
  Product1/1 -> "pdot qdot rdot "/1, " "/1
  Product2/1 -> Add/1
  Add/1 -> 3x3 Cross Product/2
  [hrw] -> Add/2

== system AOCS_FDIR/Dynamics/6DOF Model/Attitude Kinematics ==
  p q r : Inport
  Direction Cosine Matrix to Rotation Angles : sharedtransform/Direction Cosine Matrix to Rotation Angles  rotationOrder=ZYX  aMode=aMode  action=None  tolerance=eps(2)
      settings: SourceProductBaseCode=AE,PW,MT,UV,VE,VP
  Initial Quaternion : Constant  Value=q_0
  MATLAB Function1 : MATLAB Function  TreatAsAtomicUnit=on
  Product : Product  Inputs=/  Multiplication=Matrix(*)
  Product1 : Product  Multiplication=Matrix(*)
  Quaternion Evolution : Subsystem
  Quaternions to Direction Cosine Matrix : sharedtransform/Quaternions to  Direction Cosine Matrix  aMode=aMode
      settings: SourceProductBaseCode=AE,PW,MT,UV,VE,VP
  Quaternions to Rotation Angles : sharedtransform/Quaternions to Rotation Angles  rotationOrder=ZYX  aMode=aMode
      settings: SourceProductBaseCode=AE,PW,MT,UV,VE,VP
  Selector : Selector  InputPortWidth=3  IndexOptions=Index vector (dialog)  Indices=[3 2 1]  OutputSizes=1
  Selector2 : Selector  InputPortWidth=3  IndexOptions=Index vector (dialog)  Indices=[3 2 1]  OutputSizes=1
  q0 q1 q2 q3 : Integrator  InitialConditionSource=external  InitialCondition=[e0_0 e1_0 e2_0 e3_0]
  Euler_b/ECI : Outport  VectorParamsAs1DForOutWhenUnconnected=off
  DCM_b/ECI : Outport  Port=2  VectorParamsAs1DForOutWhenUnconnected=off
  q_b/ECI : Outport  Port=3  VectorParamsAs1DForOutWhenUnconnected=off
  Euler_b/LVLH : Outport  Port=4  VectorParamsAs1DForOutWhenUnconnected=off
  wires:
  p q r/1 -> Quaternion Evolution/1(p q r)
  Selector/1 -> Euler_b/ECI/1
  Quaternions to Direction Cosine Matrix/1 -> Product/1, DCM_b/ECI/1
  Quaternions to Rotation Angles/1 -> Selector/1
  q0 q1 q2 q3/1 -> q_b/ECI/1, Quaternions to Direction Cosine Matrix/1, Quaternions to Rotation Angles/1, Quaternion Evolution/2(q0 q1 q2 q3)
  Quaternion Evolution/1(qdot) -> q0 q1 q2 q3/1
  MATLAB Function1/1(DCM_LVLH_ECI) -> Product1/1
  Product/1 -> Product1/2
  Product1/1 -> Direction Cosine Matrix to Rotation Angles/1  "DCM_LVLH/b"
  Direction Cosine Matrix to Rotation Angles/1 -> Selector2/1
  Selector2/1 -> Euler_b/LVLH/1
  Initial Quaternion/1 -> q0 q1 q2 q3/2
  [r] -> MATLAB Function1/1(r)
  [v] -> MATLAB Function1/2(v)

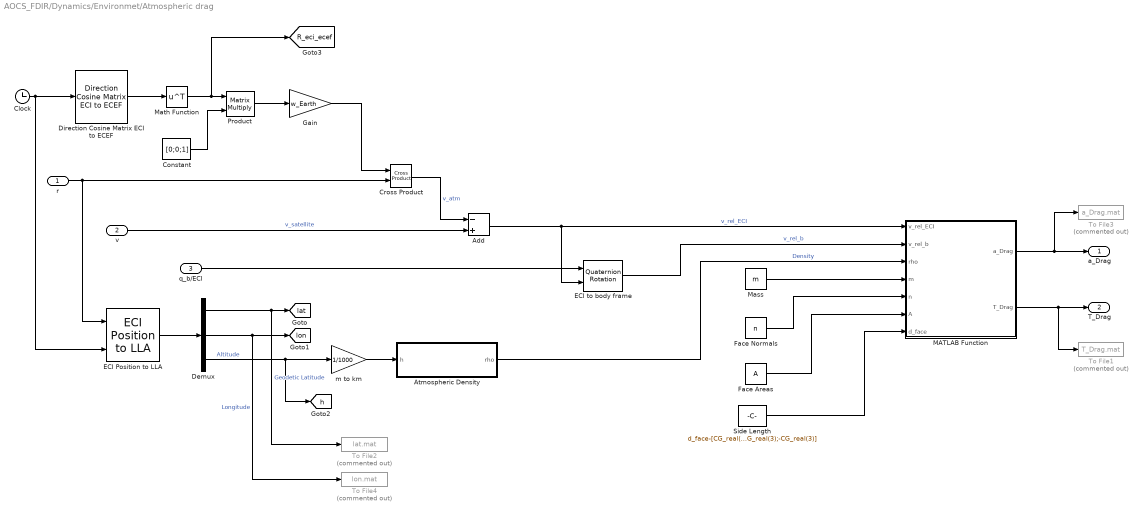
== system AOCS_FDIR/Dynamics/Environmet/Atmospheric drag ==
  r : Inport
  v : Inport  Port=2
  "q_b/ECI " : Inport  Port=3
  Add : Sum  Inputs=-+
  Atmospheric Density : MATLAB Function  TreatAsAtomicUnit=on
  Clock : Clock
  Constant : Constant  Value=[0;0;1]
  Cross Product : vrlib/Utilities/Cross Product
  Demux : Demux  Outputs=3
  Direction Cosine Matrix ECI to ECEF : aerolibtransform2/Direction Cosine Matrix ECI to ECEF  red=IAU-2000/2006  year=2019  month=March  day=1  hour=12  min=00  sec=00  deltaT=Sec  errorflag=Warning  extraparamflag=off
      settings: AttributesFormatString=%<red>  SourceProductBaseCode=AE
  ECI Position to LLA : aerolibtransform2/ECI Position to LLA  red=IAU-2000/2006  year=2019  month=March  day=1  hour=12  min=00  sec=00  deltaT=Sec  errorflag=Warning  extraparamflag=off  eunits=Metric (MKS)  earthmodel=WGS84  flat=1/298.257223563  eqradius=6378137
      settings: AttributesFormatString=%<red>  SourceProductBaseCode=AE
  ECI to body frame : aerolibutil/Quaternion Rotation
  Face Areas : Constant  Value=A
  Face Normals : Constant  Value=n
  Gain : Gain  Gain=w_Earth
  MATLAB Function : MATLAB Function  TreatAsAtomicUnit=on
  Mass : Constant  Value=m
  Math Function : Math  Operator=transpose  SignedPower=on  SaturateOnIntegerOverflow=on
  Product : Product  Multiplication=Matrix(*)
  Side Length : Constant  Value=d_face-[CG_real(1);-CG_real(1);CG_real(2);-CG_real(2);CG_real(3);-CG_real(3)]
  To File1 : ToFile  Commented=on  Filename=T_Drag.mat  MatrixName=T_Drag
  To File2 : ToFile  Commented=on  Filename=lat.mat  MatrixName=lat
  To File3 : ToFile  Commented=on  Filename=a_Drag.mat  MatrixName=a_Drag
  To File4 : ToFile  Commented=on  Filename=lon.mat  MatrixName=lon
  m to km : Gain  Gain=1/1000
  a_Drag : Outport  VectorParamsAs1DForOutWhenUnconnected=off
  T_Drag : Outport  Port=2  VectorParamsAs1DForOutWhenUnconnected=off
  tag scope: R_eci_ecef=global, h=global, lat=global, lon=global
  wires:
  Direction Cosine Matrix ECI to ECEF/1 -> Math Function/1
  Constant/1 -> Product/2
  Product/1 -> Gain/1
  Gain/1 -> Cross Product/1
  Cross Product/1 -> Add/1  "v_atm"
  v/1 -> Add/2  "v_satellite"
  Add/1 -> ECI to body frame/2, MATLAB Function/1(v_rel_ECI)  "v_rel_ECI"
  Demux/2 -> To File4/1, [lon]  "Longitude"
  ECI Position to LLA/1 -> Demux/1
  Demux/1 -> To File2/1, [lat]  "Geodetic Latitude"
  r/1 -> ECI Position to LLA/1, Cross Product/2
  m to km/1 -> Atmospheric Density/1(h)
  Atmospheric Density/1(rho) -> MATLAB Function/3(rho)  "Density"
  Clock/1 -> ECI Position to LLA/2, Direction Cosine Matrix ECI to ECEF/1
  "q_b/ECI "/1 -> ECI to body frame/1
  ECI to body frame/1 -> MATLAB Function/2(v_rel_b)  "v_rel_b"
  MATLAB Function/1(a_Drag) -> To File3/1, a_Drag/1
  MATLAB Function/2(T_Drag) -> To File1/1, T_Drag/1
  Face Normals/1 -> MATLAB Function/5(n)
  Face Areas/1 -> MATLAB Function/6(A)
  Mass/1 -> MATLAB Function/4(m)
  Side Length/1 -> MATLAB Function/7(d_face)
  Demux/3 -> m to km/1, [h]  "Altitude"
  Math Function/1 -> [R_eci_ecef], Product/1

== system AOCS_FDIR/Dynamics/Environmet/Gravity Gradient Torque ==
  "r " : Inport
  "q_b/ECI " : Inport  Port=2
  3x3 Cross Product : sharedutil/3x3 Cross Product  aMode=aMode
      settings: SourceProductBaseCode=AE,PW,MT,UV,VE,VP
  Constant : Constant  Value=-5/2
  Dot Product : DotProduct  InputSameDT=on  OutDataTypeStr=Inherit: Inherit via internal rule
  ECI to body frame : aerolibutil/Quaternion Rotation
  Gain : Gain  Gain=3*mu
  Inertia Matrix : Constant  Value=I_real
  Math Function : Math  Operator=pow  SignedPower=on  SaturateOnIntegerOverflow=on
  Product : Product  Multiplication=Matrix(*)
  Product1 : Product
  Scope : Scope
  To File3 : ToFile  Commented=on  Filename=T_GG.mat  MatrixName=T_GG
  T_GG : Outport  VectorParamsAs1DForOutWhenUnconnected=off
  wires:
  ECI to body frame/1 -> Dot Product/2, Dot Product/1, 3x3 Cross Product/1, Product/2  "r_body"
  Inertia Matrix/1 -> Product/1
  Dot Product/1 -> Math Function/1
  Constant/1 -> Math Function/2
  Math Function/1 -> Gain/1
  3x3 Cross Product/1 -> Product1/2
  Gain/1 -> Product1/1
  Product1/1 -> To File3/1, T_GG/1, Scope/1
  "q_b/ECI "/1 -> ECI to body frame/1
  "r "/1 -> ECI to body frame/2
  Product/1 -> 3x3 Cross Product/2

== system AOCS_FDIR/Dynamics/Environmet/J2 Perturbation  ==
  r : Inport
  Constant : Constant  Value=3*J2*mu*Re^2/2
  Constant1 : Constant  Value=5
  Constant2 : Constant
  Constant3 : Constant  Value=3
  Demux : Demux  Outputs=3
  Divide : Product  Inputs=/*
  Divide1 : Product  Inputs=*/
  Dot Product : DotProduct  InputSameDT=on  OutDataTypeStr=Inherit: Inherit via internal rule
  Gain : Gain  Gain=5
  Math Function : Math  Operator=pow  SignedPower=on  SaturateOnIntegerOverflow=on
  Math Function1 : Math  Operator=square  SignedPower=on  SaturateOnIntegerOverflow=on
  Mux : Mux  Inputs=3
  Product{,1..3} (4 alike) : Product
  Sqrt : Sqrt  SaturateOnIntegerOverflow=on
  Sum : Sum  Inputs=|+-
  Sum1 : Sum  Inputs=|+-
  To File3 : ToFile  Commented=on  Filename=a_J2.mat  MatrixName=a_J2
  a_J2 : Outport  VectorParamsAs1DForOutWhenUnconnected=off
  wires:
  r/1 -> Dot Product/1, Dot Product/2, Demux/1
  Dot Product/1 -> Sqrt/1, Divide1/2  "R^2"
  Sqrt/1 -> Math Function/1  "R"
  Constant1/1 -> Math Function/2
  Demux/1 -> Product/1  "x"
  Demux/2 -> Product1/1  "y"
  Demux/3 -> Product2/2, Math Function1/1  "z"
  Constant/1 -> Divide/2
  Math Function/1 -> Divide/1  "R^5"
  Math Function1/1 -> Gain/1
  Gain/1 -> Divide1/1
  Divide1/1 -> Sum/1, Sum1/1
  Constant2/1 -> Sum/2
  Sum/1 -> Product1/2, Product/2
  Constant3/1 -> Sum1/2
  Sum1/1 -> Product2/1
  Divide/1 -> Product3/2
  Product3/1 -> To File3/1, a_J2/1
  Product/1 -> Mux/1
  Product1/1 -> Mux/2
  Product2/1 -> Mux/3
  Mux/1 -> Product3/1

== system AOCS_FDIR/Dynamics/Environmet/Magnetic Torque ==
  q_b/ECI : Inport
  3x3 Cross Product : sharedutil/3x3 Cross Product  aMode=aMode
      settings: SourceProductBaseCode=AE,PW,MT,UV,VE,VP
  Constant4 : Constant  Value=Dipole_SC
  Direction Cosine Matrix ECEF to NED : aerolibtransform2/Direction Cosine Matrix ECEF to NED
      settings: SourceProductBaseCode=AE
  ECI to body frame : aerolibutil/Quaternion Rotation
  International Geomagnetic Reference Field 12 : aerolibobsolete/International Geomagnetic Reference Field 12  units=Metric (MKS)  time_in=off  month=March  day=1  year=2019  action=Warning  sv_out=off
      settings: SourceProductBaseCode=AE
  Matrix Multiply : Product  Multiplication=Matrix(*)
  Matrix Multiply1 : Product  Multiplication=Matrix(*)
  Mux : Mux  Inputs=2
  Scope : Scope
  Scope1 : Scope
  Terminator{,1..3} (4 alike) : Terminator
  To File1 : ToFile  Commented=on  Filename=B.mat  MatrixName=B
  To File2 : ToFile  Commented=on  Filename=B_b.mat  MatrixName=B_b
  To File3 : ToFile  Commented=on  Filename=T_mag.mat  MatrixName=T_mag
  Transpose : Math  Operator=transpose  SignedPower=on  SaturateOnIntegerOverflow=on
  nT to T : Gain  Gain=1e-9
  T_Mag : Outport  VectorParamsAs1DForOutWhenUnconnected=off
  tag scope: B_b=global
  wires:
  nT to T/1 -> To File1/1, ECI to body frame/2
  ECI to body frame/1 -> To File2/1, [B_b], 3x3 Cross Product/2  "Magnetic Field in Body Axis"
  q_b/ECI/1 -> ECI to body frame/1
  3x3 Cross Product/1 -> To File3/1, T_Mag/1, Scope/1
  Constant4/1 -> 3x3 Cross Product/1
  [lat] -> Mux/1, International Geomagnetic Reference Field 12/2
  [lon] -> Mux/2, International Geomagnetic Reference Field 12/3
  International Geomagnetic Reference Field 12/5 -> Terminator/1
  International Geomagnetic Reference Field 12/4 -> Terminator1/1
  International Geomagnetic Reference Field 12/3 -> Terminator2/1
  International Geomagnetic Reference Field 12/2 -> Terminator3/1
  Mux/1 -> Direction Cosine Matrix ECEF to NED/1
  [h] -> International Geomagnetic Reference Field 12/1
  Direction Cosine Matrix ECEF to NED/1 -> Transpose/1
  Transpose/1 -> Matrix Multiply/2
  [R_eci_ecef] -> Matrix Multiply/1
  Matrix Multiply/1 -> Matrix Multiply1/1
  International Geomagnetic Reference Field 12/1 -> Matrix Multiply1/2
  Matrix Multiply1/1 -> Scope1/1, nT to T/1
